simulink model "GMAW"  (R2021a)
settings: Solver=VariableStepAuto  StartTime=0.0  StopTime=3  RelTol=1e-3
libraries: pid_lib x1
settings Model: Creator=giulio  LastModifiedBy=giulio
settings DebuggingCC: UnderSpecifiedDimensionMsg=warning

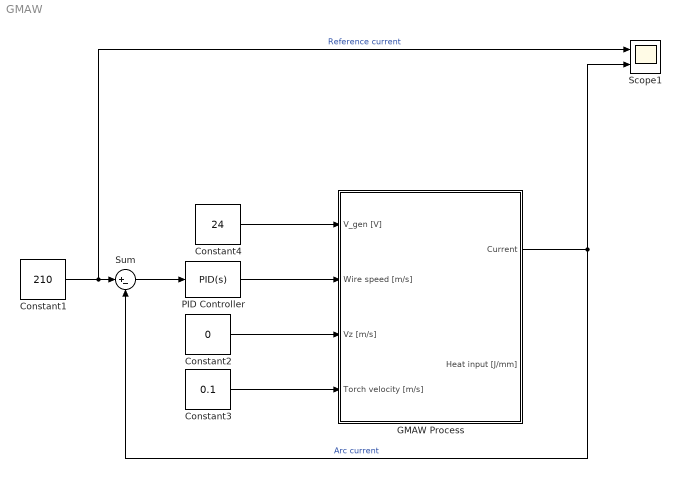
== system GMAW ==
  Constant1 : Constant  Value=210
  Constant2 : Constant  Value=0
  Constant3 : Constant  Value=0.1
  Constant4 : Constant  Value=24
  GMAW Process : Subsystem  mask(Gas Metal Arc Welding dynamic model){ls0=0.02, Rgen=0.0068, V0=12, Rarc=0.0237, Ea=400, L=3.06*10e-4, Rho=0.43, d=0.001, C1=3.3*10^-10, C2=0.78*10^-10}
      mask prompts: ls0 "Initial stick out [m]"; Rgen "Welding machine resistance [Ohm]"; V0 "Anode-catode drop [V]"; Rarc "Arc resistance [Ohm]"; Ea "Electriec field drop constant [V/m]"; L "Equivalent circuit inductance [H]"; Rho "WIre resistivity [Ohm/m]"; d "Wire diameter [m]"; C1 "Arc heating constant"; C2 "Joule heating constant"
      mask DialogControl Container3 Prompt: Electrical parameters
      mask DialogControl Container4 Prompt: Wire parameters
      mask DialogControl Container5 Prompt: Melting parameters
  PID Controller : pid_lib/PID Controller  Controller=PID  Form=Parallel  TimeDomain=Continuous-time  UseExternalTs=off  SampleTime=-1  IntegratorMethod=Forward Euler  FilterMethod=Forward Euler  ControllerParametersSource=internal  P=0.02  I=0.01  D=0  UseFilter=on  N=0  TunerSelectOption=Transfer Function Based (PID Tuner App)  InitialConditionSource=internal  InitialConditionForIntegrator=0  InitialConditionForFilter=0  DifferentiatorICPrevScaledInput=0  ExternalReset=none  TrackingMode=off  Kt=1  LimitOutput=on  SatLimitsSource=internal  UpperSaturationLimit=0.15  LowerSaturationLimit=-0.15  LinearizeAsGain=on  AntiWindupMode=none  Kb=1  POutMin=[]  POutMax=[]  IOutMin=[]  IOutMax=[]  DOutMin=[]  DOutMax=[]  NOutMin=[]  NOutMax=[]  SumOutMin=[]  SumOutMax=[]  SaturationOutMin=[]  SaturationOutMax=[]  PParamMin=[]  PParamMax=[]  IParamMin=[]  IParamMax=[]  DParamMin=[]  DParamMax=[]  NParamMin=[]  NParamMax=[]  KbParamMin=[]  KbParamMax=[]  KtParamMin=[]  KtParamMax=[]  KbOutMin=[]  KbOutMax=[]  KtOutMin=[]  KtOutMax=[]  IntegratorOutMin=[]  IntegratorOutMax=[]  FilterOutMin=[]  FilterOutMax=[]  SumI1OutMin=[]  SumI1OutMax=[]  SumI2OutMin=[]  SumI2OutMax=[]  SumI3OutMin=[]  SumI3OutMax=[]  SumI4OutMin=[]  SumI4OutMax=[]  SumDOutMin=[]  SumDOutMax=[]  DifferentiatorOutMin=[]  DifferentiatorOutMax=[]  FilterDiffOutCoefMin=[]  FilterDiffOutCoefMax=[]  ReciprocalOutMin=[]  ReciprocalOutMax=[]  SumDenOutMin=[]  SumDenOutMax=[]  SumNumOutMin=[]  SumNumOutMax=[]  DivideOutMin=[]  DivideOutMax=[]  UdiffTsProdOutMin=[]  UdiffTsProdOutMax=[]  NTsProdOutMin=[]  NTsProdOutMax=[]  UintegralTsProdOutMin=[]  UintegralTsProdOutMax=[]  UngainTsProdOutMin=[]  UngainTsProdOutMax=[]  IntegratorContinuousStateAttributes=''  IntegratorStateMustResolveToSignalObject=off  IntegratorRTWStateStorageClass=Auto  FilterContinuousStateAttributes=''  FilterStateMustResolveToSignalObject=off  FilterRTWStateStorageClass=Auto  ParallelPVariant=InternalParameters  IdealPVariant=Disabled  IVariant=InternalParameters  DVariant=InternalParameters  IntegratorVariant=Continuous  SatVariant=Enabled  AWVariant=Passthrough  PCopyVariant=Disabled  TRVariant=Disabled  FdbkBlocksVariant=Forward  IdealPFdbkVariant=Disabled  SatFdbkVariant=Disabled  DerivativeFilterVariant=ContFilter  NVariant=InternalParameters  NCopyVariant=Disabled  FilterICVariant=InternalICsFilter  IntegratorICVariant=InternalICs  ExternalResetVariant=Disabled  TRSumVariant=Passthrough  SumFdbkVariant=Disabled  SumVariant=Sum_PID  TsampFilterVariant=InternalTs  TsampNgainVariant=Passthrough  TsampIntegralVariant=Passthrough  ExternalSaturationOutDataTypeStr=Inherit: Same as second input
  Scope1 : Scope  NumInputPorts=2
  Sum : Sum  Inputs=|+-
  wires:
  GMAW Process/1(Current) -> Sum/2, Scope1/2  "Arc current"
  Constant2/1 -> GMAW Process/3(Vz [m/s])
  Constant3/1 -> GMAW Process/4(Torch velocity [m/s])
  Constant4/1 -> GMAW Process/1(V_gen [V])
  PID Controller/1 -> GMAW Process/2(Wire speed [m/s])
  Sum/1 -> PID Controller/1
  Constant1/1 -> Scope1/1, Sum/1  "Reference current"

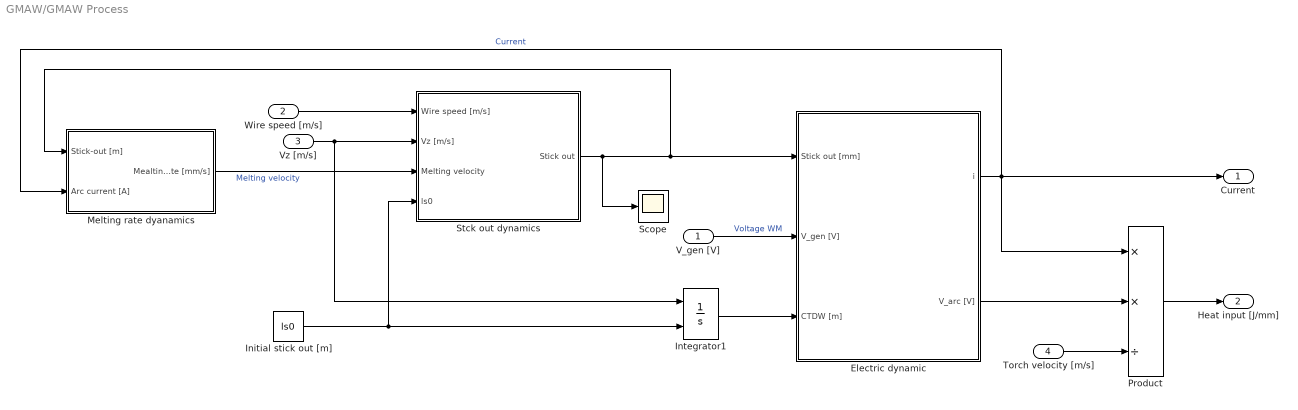
== system GMAW/GMAW Process ==
  V_gen [V] : Inport
  Wire speed [m/s] : Inport  Port=2
  Vz [m/s] : Inport  Port=3
  Torch velocity [m/s] : Inport  Port=4
  Electric dynamic : Subsystem
  Initial stick out [m] : Constant  Value=ls0
  Integrator1 : Integrator  InitialConditionSource=external
  Melting rate dyanamics : Subsystem
  Product : Product  Inputs=**/
  Scope : Scope
  Stck out dynamics : Subsystem
  Current : Outport
  Heat input [J/mm] : Outport  Port=2
  wires:
  V_gen [V]/1 -> Electric dynamic/2(V_gen [V])  "Voltage WM"
  Electric dynamic/1(i) -> Product/1, Melting rate dyanamics/2(Arc current [A]), Current/1  "Current"
  Product/1 -> Heat input [J/mm]/1
  Electric dynamic/2(V_arc [V]) -> Product/2
  Torch velocity [m/s]/1 -> Product/3
  Initial stick out [m]/1 -> Integrator1/2, Stck out dynamics/4(ls0)
  Integrator1/1 -> Electric dynamic/3(CTDW [m])
  Stck out dynamics/1(Stick out) -> Scope/1, Melting rate dyanamics/1(Stick-out [m]), Electric dynamic/1("Stick out [mm] ")
  Wire speed [m/s]/1 -> Stck out dynamics/1(Wire speed [m/s])
  Vz [m/s]/1 -> Integrator1/1, Stck out dynamics/2(Vz [m/s])
  Melting rate dyanamics/1(Mealting rate [mm/s]) -> Stck out dynamics/3(Melting velocity)  "Melting velocity"

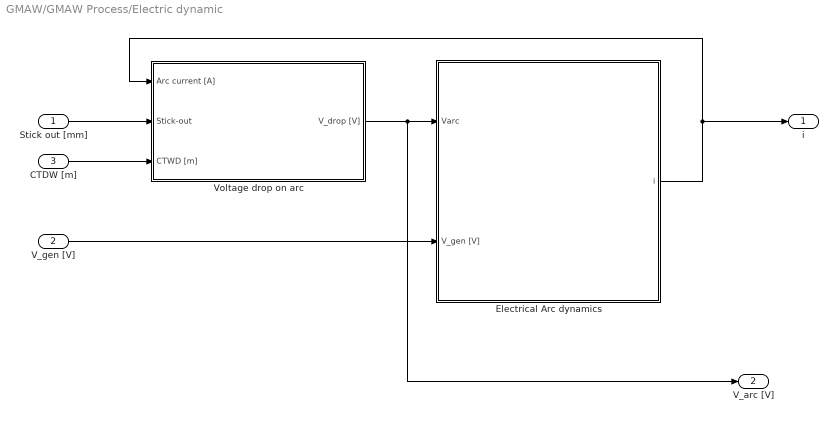
== system GMAW/GMAW Process/Electric dynamic ==
  "Stick out [mm] " : Inport
  V_gen [V] : Inport  Port=2
  CTDW [m] : Inport  Port=3
  Electrical Arc dynamics : Subsystem
  Voltage drop on arc : Subsystem
  i : Outport
  V_arc [V] : Outport  Port=2
  wires:
  "Stick out [mm] "/1 -> Voltage drop on arc/2(Stick-out)
  Electrical Arc dynamics/1(i) -> i/1, Voltage drop on arc/1(Arc current [A])
  V_gen [V]/1 -> Electrical Arc dynamics/2(V_gen [V])
  CTDW [m]/1 -> Voltage drop on arc/3(CTWD [m])
  Voltage drop on arc/1(V_drop [V]) -> V_arc [V]/1, Electrical Arc dynamics/1(Varc)

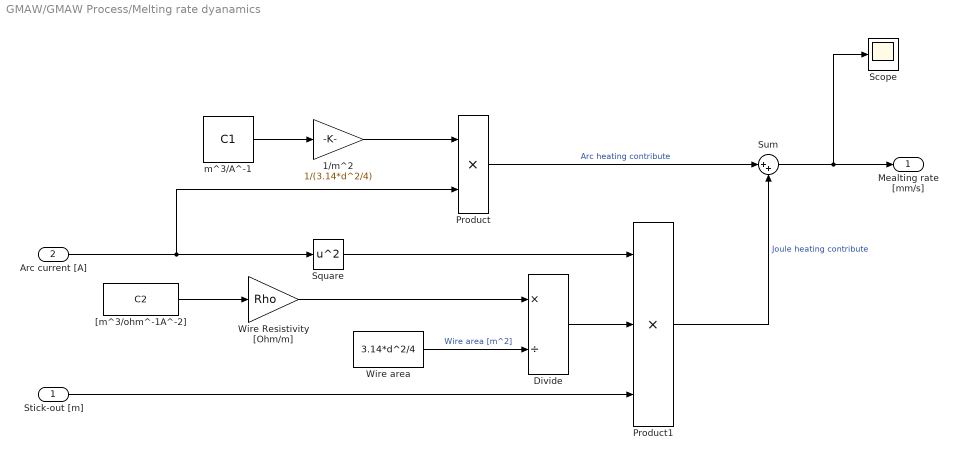
== system GMAW/GMAW Process/Melting rate dyanamics ==
  Stick-out [m] : Inport
  Arc current [A] : Inport  Port=2
  1/m^2 : Gain  Gain=1/(3.14*d^2/4)
  Divide : Product  Inputs=*/
  Product : Product
  Product1 : Product  Inputs=3
  Scope : Scope
  Square : Math  Operator=square  SaturateOnIntegerOverflow=on
  Sum : Sum  Inputs=|++
  Wire Resistivity [Ohm/m] : Gain  Gain=Rho
  Wire area : Constant  Value=3.14*d^2/4
  "[m^3/ohm^-1A^-2]" : Constant  Value=C2
  m^3/A^-1 : Constant  Value=C1
  Mealting rate [mm/s] : Outport
  wires:
  Product/1 -> Sum/1  "Arc heating contribute"
  Divide/1 -> Product1/2
  1/m^2/1 -> Product/1
  Wire Resistivity [Ohm/m]/1 -> Divide/1
  "[m^3/ohm^-1A^-2]"/1 -> Wire Resistivity [Ohm/m]/1
  m^3/A^-1/1 -> 1/m^2/1
  Square/1 -> Product1/1
  Stick-out [m]/1 -> Product1/3
  Arc current [A]/1 -> Product/2, Square/1
  Wire area/1 -> Divide/2  "Wire area [m^2]"
  Product1/1 -> Sum/2  "Joule heating contribute"
  Sum/1 -> Scope/1, Mealting rate [mm/s]/1

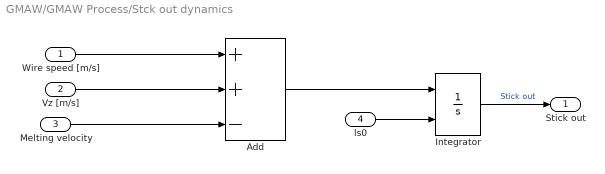
== system GMAW/GMAW Process/Stck out dynamics ==
  Wire speed [m/s] : Inport
  Vz [m/s] : Inport  Port=2
  Melting velocity : Inport  Port=3
  ls0 : Inport  Port=4
  Add : Sum  Inputs=++-
  Integrator : Integrator  InitialConditionSource=external
  Stick out : Outport
  wires:
  ls0/1 -> Integrator/2
  Vz [m/s]/1 -> Add/2
  Add/1 -> Integrator/1
  Integrator/1 -> Stick out/1  "Stick out"
  Wire speed [m/s]/1 -> Add/1
  Melting velocity/1 -> Add/3

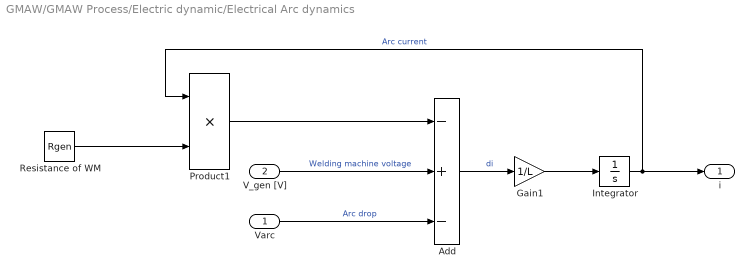
== system GMAW/GMAW Process/Electric dynamic/Electrical Arc dynamics ==
  Varc : Inport
  V_gen [V] : Inport  Port=2
  Add : Sum  Inputs=-+-
  Gain1 : Gain  Gain=1/L
  Integrator : Integrator
  Product1 : Product
  Resistance of WM : Constant  Value=Rgen
  i : Outport
  wires:
  Varc/1 -> Add/3  "Arc drop"
  V_gen [V]/1 -> Add/2  "Welding machine voltage"
  Integrator/1 -> Product1/1, i/1  "Arc current"
  Add/1 -> Gain1/1  "di"
  Gain1/1 -> Integrator/1
  Product1/1 -> Add/1
  Resistance of WM/1 -> Product1/2

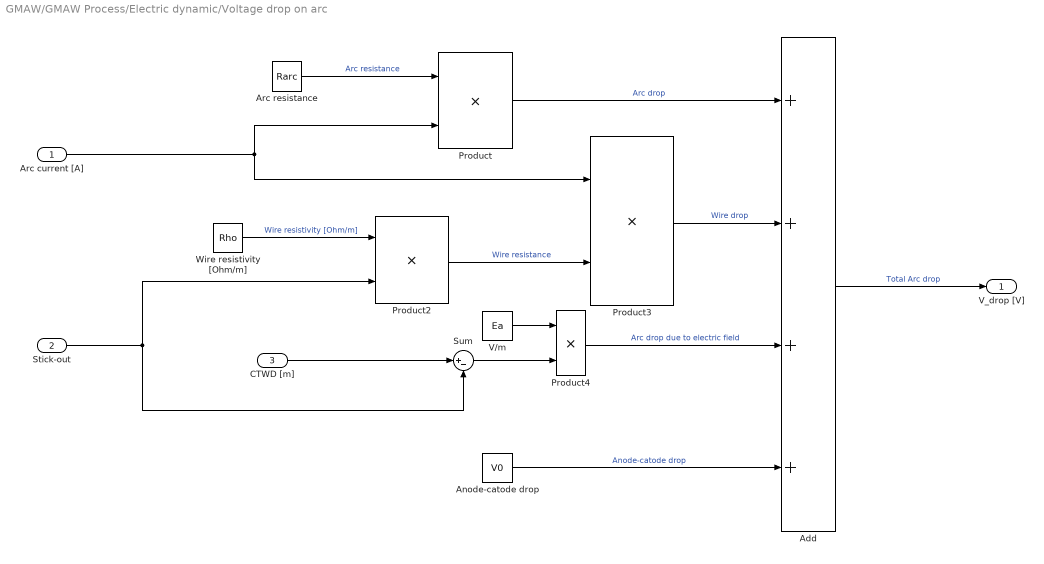
== system GMAW/GMAW Process/Electric dynamic/Voltage drop on arc ==
  Arc current [A] : Inport
  Stick-out : Inport  Port=2
  CTWD [m] : Inport  Port=3
  Add : Sum  Inputs=++++
  Anode-catode drop : Constant  Value=V0
  Arc resistance : Constant  Value=Rarc
  Product{,2..4} (4 alike) : Product
  Sum : Sum  Inputs=|+-
  V/m : Constant  Value=Ea
  Wire resistivity [Ohm/m] : Constant  Value=Rho
  V_drop [V] : Outport
  wires:
  Product4/1 -> Add/3  "Arc drop due to electric field"
  Wire resistivity [Ohm/m]/1 -> Product2/1  "Wire resistivity [Ohm/m]"
  Product/1 -> Add/1  "Arc drop"
  Add/1 -> V_drop [V]/1  "Total Arc drop"
  Product3/1 -> Add/2  "Wire drop"
  Product2/1 -> Product3/2  "Wire resistance"
  Stick-out/1 -> Sum/2, Product2/2
  Arc current [A]/1 -> Product3/1, Product/2
  Sum/1 -> Product4/2
  V/m/1 -> Product4/1
  Anode-catode drop/1 -> Add/4  "Anode-catode drop"
  Arc resistance/1 -> Product/1  "Arc resistance"
  CTWD [m]/1 -> Sum/1
